simulink model "simPos"  (R2016b)
settings: Solver=ode45  StartTime=0.0  StopTime=60  RelTol=1e-3  EnableMultiTasking=on
values from neighbouring files (symbols this model uses):
  K0 = 256.141887526    [controller.mat]
  KVmax = 1128.52050948    [controller.mat]
undefined symbols (not defined in the file or in its folder): Arm, Fmax, Kd, M, motorDeadZone, sensorPeriod, Vmax
libraries: simulink x2, cstblocks x1
settings Model: Creator=Cassandra  LastModifiedBy=Cassandra
settings DataIOCC: LimitDataPoints=on  SaveFormat=Array
settings OptimizationCC: LifeSpan=inf
settings DebuggingCC: MaxConsecutiveZCsMsg=none  SFUnexpectedBacktrackingDiag=warning  SFNoUnconditionalDefaultTransitionDiag=warning  SFExecutionAtInitializationDiag=none
settings HardwareCC: ProdBitPerPointer=32  ProdBitPerSizeT=32  ProdBitPerPtrDiffT=32  ProdLargestAtomicFloat=None  ProdIntDivRoundTo=Undefined  ProdEndianess=Unspecified  ProdWordSize=32  ProdHWDeviceType=32-bit Generic
settings ModelReferenceCC: PropagateSignalLabelsOutOfModel=off
settings GRTTargetCC: TargetLangStandard=C89/C90 (ANSI)  GeneratePreprocessorConditionals=Disable all
settings ConfigComp: CovMetricSettings=dw  CovHtmlReporting=on  CovSaveCumulativeToWorkspaceVar=on  CovSaveSingleToWorkspaceVar=on  CovExternalEMLEnable=off

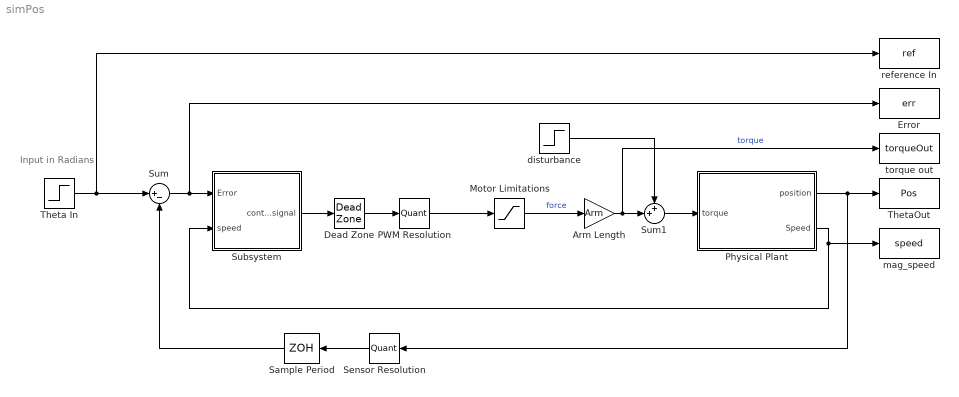
== system simPos ==
  note: Input in Radians
  Arm Length : Gain  Gain=Arm
  Dead Zone : DeadZone  LowerValue=-motorDeadZone  UpperValue=motorDeadZone  SaturateOnIntegerOverflow=on
  Error : ToWorkspace  VariableName=err  SaveFormat=Timeseries  SampleTime=-1
  Motor Limitations : Saturate  UpperLimit=Fmax  LowerLimit=-Fmax
  PWM Resolution : Quantizer  QuantizationInterval=motorResolution
  Physical Plant : Subsystem
  Sample Period : ZeroOrderHold  SampleTime=sensorPeriod
  Sensor Resolution : Quantizer  QuantizationInterval=sensorResolution
  Subsystem : Subsystem
  Sum : Sum  Inputs=|+-
  Sum1 : Sum  Inputs=++|
  Theta In : Step  After=pi/2  SampleTime=0
  ThetaOut : ToWorkspace  VariableName=Pos  SaveFormat=Timeseries  SampleTime=-1
  disturbance : Step  Time=20  After=5  SampleTime=0
  mag_speed : ToWorkspace  VariableName=speed  SaveFormat=Timeseries  SampleTime=-1
  reference In : ToWorkspace  VariableName=ref  SaveFormat=Timeseries  SampleTime=-1
  torque out : ToWorkspace  VariableName=torqueOut  SaveFormat=Timeseries  SampleTime=-1
  wires:
  Theta In/1 -> reference In/1, Sum/1
  PWM Resolution/1 -> Motor Limitations/1
  Sensor Resolution/1 -> Sample Period/1
  Physical Plant/1(position) -> ThetaOut/1, Sensor Resolution/1
  Physical Plant/2(Speed) -> Subsystem/2(speed), mag_speed/1
  Sum/1 -> Subsystem/1(Error), Error/1
  Sample Period/1 -> Sum/2
  Motor Limitations/1 -> Arm Length/1  "force"
  Dead Zone/1 -> PWM Resolution/1
  Subsystem/1(control signal) -> Dead Zone/1
  Arm Length/1 -> torque out/1, Sum1/2  "torque"
  Sum1/1 -> Physical Plant/1(torque)
  disturbance/1 -> Sum1/1

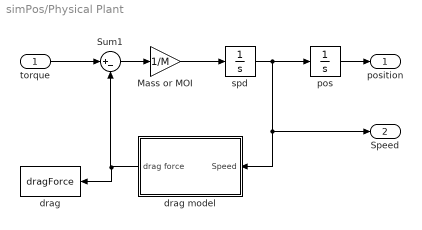
== system simPos/Physical Plant ==
  torque : Inport
  Mass or MOI : Gain  Gain=1/M
  Sum1 : Sum  Inputs=|+-
  drag : ToWorkspace  VariableName=dragForce  SaveFormat=Timeseries  SampleTime=-1
  drag model : Subsystem
  pos : Integrator
  spd : Integrator
  position : Outport
  Speed : Outport  Port=2
  wires:
  spd/1 -> pos/1, drag model/1(Speed), Speed/1
  Mass or MOI/1 -> spd/1
  pos/1 -> position/1
  Sum1/1 -> Mass or MOI/1
  drag model/1(drag force) -> Sum1/2, drag/1
  torque/1 -> Sum1/1

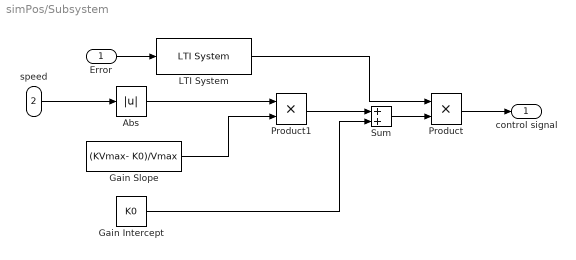
== system simPos/Subsystem ==
  Error : Inport
  speed : Inport  Port=2
  Abs : Abs
  Gain Intercept : Constant  Value=K0
  Gain Slope : Constant  Value=(KVmax- K0)/Vmax
  LTI System : cstblocks/LTI System  sys=C0  IC=[]
  Product : Product
  Product1 : Product
  Sum : Sum
  control signal : Outport
  wires:
  speed/1 -> Abs/1
  Abs/1 -> Product1/1
  Product/1 -> control signal/1
  Sum/1 -> Product/2
  Product1/1 -> Sum/1
  LTI System/1 -> Product/1
  Error/1 -> LTI System/1
  Gain Slope/1 -> Product1/2
  Gain Intercept/1 -> Sum/2

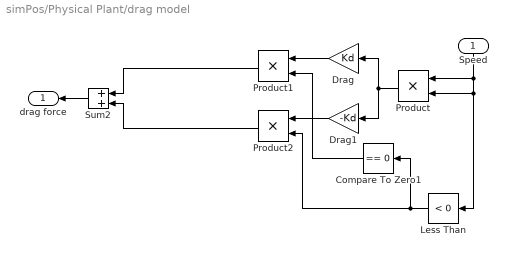
== system simPos/Physical Plant/drag model ==
  Speed : Inport
  Compare To Zero1 : simulink/Logic and Bit Operations/Compare To Zero  relop===  OutDataTypeStr=boolean
  Drag : Gain  Gain=Kd
  Drag1 : Gain  Gain=-Kd
  Less Than : simulink/Logic and Bit Operations/Compare To Zero  relop=<  OutDataTypeStr=boolean
  Product : Product
  Product1 : Product
  Product2 : Product
  Sum2 : Sum  Inputs=+|+
  drag force : Outport
  wires:
  Speed/1 -> Product/1, Less Than/1, Product/2
  Drag1/1 -> Product2/1
  Compare To Zero1/1 -> Product1/2
  Product1/1 -> Sum2/1
  Drag/1 -> Product1/1
  Sum2/1 -> drag force/1
  Product/1 -> Drag1/1, Drag/1
  Product2/1 -> Sum2/2
  Less Than/1 -> Product2/2, Compare To Zero1/1
